simulink model "OES_roe"  (R2018b)
settings: configuration reference "Configuration" (kept outside this file)
undefined symbols (not defined in the file): roe, sats, TimeStep
settings Model: Creator=Ethan  LastModifiedBy=Ethan
settings ConfigSetRef: SourceLocation=Base Workspace

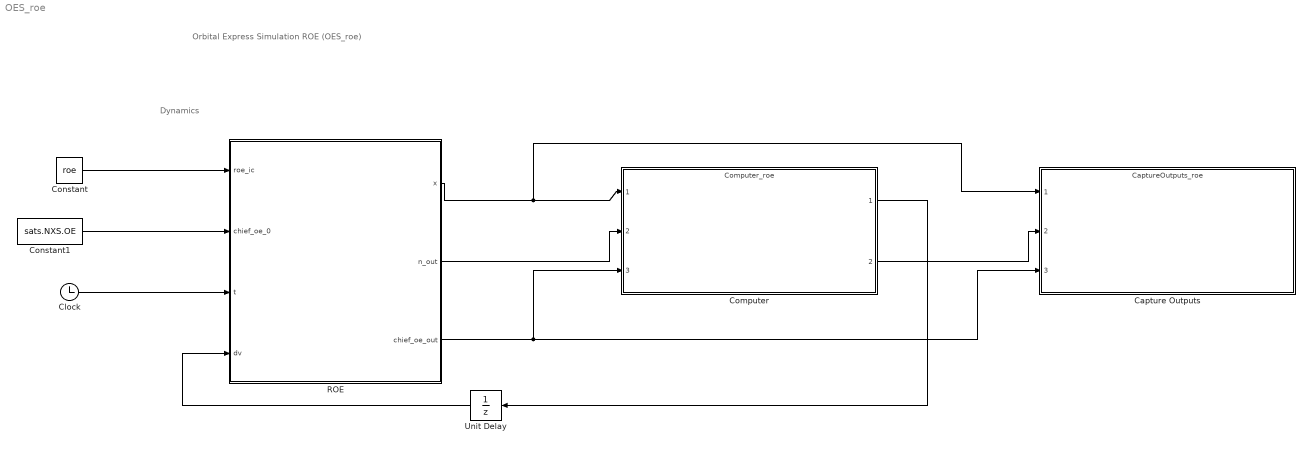
== system OES_roe ==
  note: Dynamics
  note: Orbital Express Simulation ROE (OES_roe)
  Capture Outputs : ModelReference  ModelNameDialog=CaptureOutputs_roe.slx  ParameterArgumentNames=CON  ParameterArgumentValues=CON  UsingDefaultArgumentValue=0  SimulationMode=Normal  ModelReferenceVersion=1.86
  Clock : Clock
  Computer : ModelReference  ModelNameDialog=Computer_roe.slx  ParameterArgumentNames=CON  ParameterArgumentValues=CON  UsingDefaultArgumentValue=0  SimulationMode=Normal  ModelReferenceVersion=1.262
  Constant : Constant  Value=roe  OutDataTypeStr=Bus: Bus_roe
  Constant1 : Constant  Value=sats.NXS.OE  OutDataTypeStr=Bus: Bus_OE
  ROE : MATLAB Function  TreatAsAtomicUnit=on  SystemSampleTime=TimeStep
  Unit Delay : UnitDelay  SampleTime=-1
  wires:
  Clock/1 -> ROE/3(t)
  ROE/1(x) -> Capture Outputs/1, Computer/1
  ROE/2(n_out) -> Computer/2
  Computer/2 -> Capture Outputs/2
  Computer/1 -> Unit Delay/1
  Unit Delay/1 -> ROE/4(dv)
  Constant/1 -> ROE/1(roe_ic)
  Constant1/1 -> ROE/2(chief_oe_0)
  ROE/3(chief_oe_out) -> Computer/3, Capture Outputs/3

== matlab function OES_roe/ROE ==
  data: roe_ic input Bus: Bus_roe; chief_oe_0 input Bus: Bus_OE; x output; t input; dv input; CON parameter; n_out output; chief_oe_out output Bus: Bus_OE
function [x, n_out, chief_oe_out] = roe_prop(roe_ic, chief_oe_0, t, dv, CON)
persistent x0 t0 x_prev chief_oe M0 n t0_chief_prop
if isempty(x0)
    t0 = t;
    x0 = [roe_ic.adot; roe_ic.da; roe_ic.dL; roe_ic.dex; roe_ic.dey;...
        roe_ic.dix; roe_ic.diy];
    chief_oe = chief_oe_0;
    x_prev = x0;
    E0 = 2 * atan(sqrt((1-chief_oe.e)/(1+chief_oe.e)) * tand(chief_oe.nu/2));
    M0 = E0 - chief_oe.e * sin(E0);
    n = sqrt(CON.mu / chief_oe.a^3);
    t0_chief_prop = t0;
end

n_out = n;
eta = sqrt(1 - chief_oe.e^2);
gamma = CON.J2/2 * (CON.Re / chief_oe.a)^2 * (1 / eta^4);
A = roe_state_matrix(n, t - t0, chief_oe.inc, gamma, CON);


% if any(dv ~= zeros(4, 1))
%     x0(2) = x_prev(2) + 2 * dv(2) / (n * chief_oe.a);
%     x0(3) = x_prev(3) - 2 * dv(1) / (n * chief_oe.a);
%     x0(4) = x_prev(4) + dv(1) * sin(dv(4)) / (n * chief_oe.a) + ...
%         2 * dv(2) * cos(dv(4)) / (n * chief_oe.a);
%     x0(5) = x_prev(5) - dv(1) * cos(dv(4)) / (n * chief_oe.a) + ...
%         2 * dv(2) * sin(dv(4)) / (n * chief_oe.a);
%     
%     A = roe_state_matrix(n, 0, chief_oe.inc, gamma, CON);
%     x = A * x0;
%     t0 = t;
% else
    x = A * x0;
% end

M = M0 + n * (t - t0_chief_prop);
E = M2E(M, chief_oe.e, 1e-6);

chief_oe.nu = 2 * atan(sqrt((1+chief_oe.e)/(1-chief_oe.e)) * tan(E/2)) * 180 / pi;
chief_oe_out = chief_oe;

x_prev = x;
end
